simulink library "casper_library_accumulators"  (Simulink 7.0)
values from neighbouring files (symbols this model uses):
  blockCountBits = ceil(log2(numBlocks))    [readback_address_dram_vacc_mask.m]
  blockRowBits = 0    [readback_address_dram_vacc_mask.m]
libraries: xbsIndex_r4 x622, xbsReplacements_r4 x61, casper_library_misc x17, xps_library x9
(part 2 of 5)

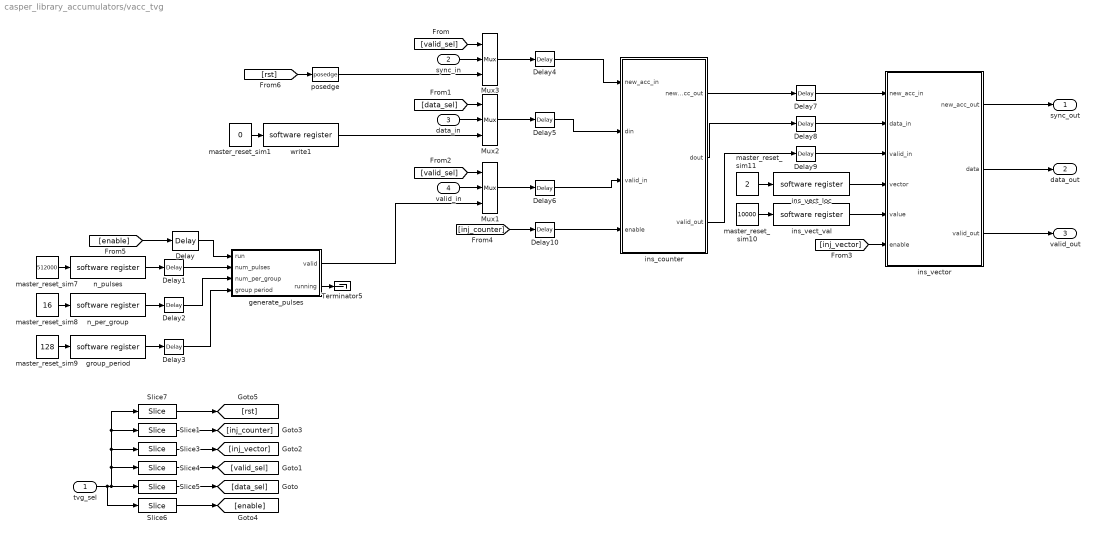
== system casper_library_accumulators/vacc_tvg ==
  tvg_sel : Inport  OutDataType=sfix(16)  OutScaling=2^0
  sync_in : Inport  Port=2  OutDataType=sfix(16)  OutScaling=2^0
  data_in : Inport  Port=3  OutDataType=sfix(16)  OutScaling=2^0
  valid_in : Inport  Port=4  OutDataType=sfix(16)  OutScaling=2^0
  Delay : xbsIndex_r4/Delay  en=off  latency=1  dbl_ovrd=off  reg_retiming=on  block_type=delay
      settings: xl_area=[0, 0, 0, 0, 0, 0, 0]
  Delay{1..10} (10 alike) : xbsIndex_r4/Delay  en=off  latency=2  dbl_ovrd=off  reg_retiming=on  block_type=delay
  Mux1 : xbsIndex_r4/Mux  inputs=2  en=off  latency=0  precision=Full  arith_type="Signed  (2's comp)"  n_bits=8  bin_pt=2  quantization=Truncate  overflow=Wrap  dbl_ovrd=off  block_type=mux
      settings: xl_area=[0, 0, 0, 0, 0, 0, 0]
  Mux2 : xbsIndex_r4/Mux  inputs=2  en=off  latency=0  precision=Full  arith_type="Signed  (2's comp)"  n_bits=8  bin_pt=2  quantization=Truncate  overflow=Wrap  dbl_ovrd=off  block_type=mux
      settings: xl_area=[0, 0, 0, 0, 0, 0, 0]
  Mux3 : xbsIndex_r4/Mux  inputs=2  en=off  latency=0  precision=Full  arith_type="Signed  (2's comp)"  n_bits=8  bin_pt=2  quantization=Truncate  overflow=Wrap  dbl_ovrd=off  block_type=mux
      settings: xl_area=[0, 0, 0, 0, 0, 0, 0]
  Slice1 : xbsIndex_r4/Slice  nbits=1  boolean_output=on  mode=Lower Bit Location + Width  bit1=0  base1=MSB of Input  bit0=4  base0=LSB of Input  dbl_ovrd=off  block_type=slice
      settings: infoedit="Extracts a given range of bits from each input sample and presents it at the output.  The output type is ordinarily unsigned with binary point at zero, but can be Boolean when the slice is one bit wide.<P><P>Hardware notes: In hardware this block costs nothing."  block_version=10.1.3
  Slice3 : xbsIndex_r4/Slice  nbits=1  boolean_output=on  mode=Lower Bit Location + Width  bit1=0  base1=MSB of Input  bit0=3  base0=LSB of Input  dbl_ovrd=off  block_type=slice
      settings: infoedit="Extracts a given range of bits from each input sample and presents it at the output.  The output type is ordinarily unsigned with binary point at zero, but can be Boolean when the slice is one bit wide.<P><P>Hardware notes: In hardware this block costs nothing."  block_version=10.1.3
  Slice4 : xbsIndex_r4/Slice  nbits=1  boolean_output=on  mode=Lower Bit Location + Width  bit1=0  base1=MSB of Input  bit0=2  base0=LSB of Input  dbl_ovrd=off  block_type=slice
      settings: infoedit="Extracts a given range of bits from each input sample and presents it at the output.  The output type is ordinarily unsigned with binary point at zero, but can be Boolean when the slice is one bit wide.<P><P>Hardware notes: In hardware this block costs nothing."  block_version=10.1.3
  Slice5 : xbsIndex_r4/Slice  nbits=1  boolean_output=on  mode=Lower Bit Location + Width  bit1=0  base1=MSB of Input  bit0=1  base0=LSB of Input  dbl_ovrd=off  block_type=slice
      settings: infoedit="Extracts a given range of bits from each input sample and presents it at the output.  The output type is ordinarily unsigned with binary point at zero, but can be Boolean when the slice is one bit wide.<P><P>Hardware notes: In hardware this block costs nothing."  block_version=10.1.3
  Slice6 : xbsIndex_r4/Slice  nbits=1  boolean_output=on  mode=Lower Bit Location + Width  bit1=0  base1=MSB of Input  bit0=0  base0=LSB of Input  dbl_ovrd=off  block_type=slice
      settings: infoedit="Extracts a given range of bits from each input sample and presents it at the output.  The output type is ordinarily unsigned with binary point at zero, but can be Boolean when the slice is one bit wide.<P><P>Hardware notes: In hardware this block costs nothing."  block_version=10.1.3
  Slice7 : xbsIndex_r4/Slice  nbits=1  boolean_output=on  mode=Lower Bit Location + Width  bit1=0  base1=MSB of Input  bit0=5  base0=LSB of Input  dbl_ovrd=off  block_type=slice
      settings: infoedit="Extracts a given range of bits from each input sample and presents it at the output.  The output type is ordinarily unsigned with binary point at zero, but can be Boolean when the slice is one bit wide.<P><P>Hardware notes: In hardware this block costs nothing."  block_version=10.1.3
  Terminator5 : Terminator
  generate_pulses : Subsystem
  group_period : xps_library/software register  Tag=xps:sw_reg  SystemSampleTime=-1  io_dir=From Processor  arith_type=Unsigned  bitwidth=32  bin_pt=0  sample_period=1  gw_name=r_4f_2x_16a_r322m_vacc_tvg0_group_period_user_data_out
      link override qdr_vacc_dram_tvg1_group_period_user_data_out: arith_type=Unsigned  n_bits=32  bin_pt=0  period=1
      link override qdr_vacc_qdr_tvg_group_period_user_data_out: arith_type=Unsigned  n_bits=32  bin_pt=0  period=1
      link override r_4f_2x_16a_r322m_vacc_tvg0_group_period_user_data_out: arith_type=Unsigned  n_bits=32  bin_pt=0  period=1
      link override test_d_v_p_10_1_new_packet_format_qdr_tvg_group_period_user_data_out: arith_type=Unsigned  n_bits=32  bin_pt=0  period=1
      link override test_qdr_vacc2_vacc_tvg_group_period_user_data_out: arith_type=Unsigned  n_bits=32  bin_pt=0  period=1
      link override test_qdr_vacc3_vacc_tvg_group_period_user_data_out: arith_type=Unsigned  n_bits=32  bin_pt=0  period=1
      link override test_qdr_vacc_qdr_tvg_group_period_user_data_out: arith_type=Unsigned  n_bits=32  bin_pt=0  period=1
      link override test_qdr_vacc_vacc_tvg_group_period_user_data_out: arith_type=Unsigned  n_bits=32  bin_pt=0  period=1
      link override test_vacc_10_1_new_pkt_form_qdr_tvg_group_period_user_data_out: arith_type=Unsigned  n_bits=32  bin_pt=0  period=1
      link override test_vacc_pkt_10_1_vacc_tvg0_group_period_user_data_out: arith_type=Unsigned  n_bits=32  bin_pt=0  period=1
      link override test_vacc_pkt_10_1_vacc_tvg_group_period_user_data_out: arith_type=Unsigned  n_bits=32  bin_pt=0  period=1
      link override xflow_sim_8a_vacc_tvg0_group_period_user_data_out: arith_type=Unsigned  n_bits=32  bin_pt=0  period=1
      link override xflow_sim_vacc_tvg0_group_period_user_data_out: arith_type=Unsigned  n_bits=32  bin_pt=0  period=1
  ins_counter : Subsystem  mask{vec_len=len}
      mask prompts: vec_len "Vector Length?"
      mask init:
      | fmtstr = sprintf('Vector Length: %d', vec_len);
      | set_param(gcb, 'AttributesFormatString', fmtstr);
      settings: AttributesFormatString=Vector Length: 139264
  ins_vect_loc : xps_library/software register  Tag=xps:sw_reg  SystemSampleTime=-1  io_dir=From Processor  arith_type=Unsigned  bitwidth=32  bin_pt=0  sample_period=1  gw_name=r_4f_2x_16a_r322m_vacc_tvg0_ins_vect_loc_user_data_out
      link override qdr_vacc_dram_tvg1_inject_vector_location_user_data_out: arith_type=Unsigned  n_bits=32  bin_pt=0  period=1
      link override qdr_vacc_qdr_tvg_inject_vector_location_user_data_out: arith_type=Unsigned  n_bits=32  bin_pt=0  period=1
      link override r_4f_2x_16a_r322m_vacc_tvg0_ins_vect_loc_user_data_out: arith_type=Unsigned  n_bits=32  bin_pt=0  period=1
      link override test_d_v_p_10_1_new_packet_format_qdr_tvg_inject_vector_location_user_data_out: arith_type=Unsigned  n_bits=32  bin_pt=0  period=1
      link override test_qdr_vacc2_vacc_tvg_ins_vect_loc_user_data_out: arith_type=Unsigned  n_bits=32  bin_pt=0  period=1
      link override test_qdr_vacc3_vacc_tvg_ins_vect_loc_user_data_out: arith_type=Unsigned  n_bits=32  bin_pt=0  period=1
      link override test_qdr_vacc_qdr_tvg_inject_vector_location_user_data_out: arith_type=Unsigned  n_bits=32  bin_pt=0  period=1
      link override test_qdr_vacc_vacc_tvg_ins_vect_loc_user_data_out: arith_type=Unsigned  n_bits=32  bin_pt=0  period=1
      link override test_vacc_10_1_new_pkt_form_qdr_tvg_inject_vector_location_user_data_out: arith_type=Unsigned  n_bits=32  bin_pt=0  period=1
      link override test_vacc_pkt_10_1_vacc_tvg0_ins_vect_loc_user_data_out: arith_type=Unsigned  n_bits=32  bin_pt=0  period=1
      link override test_vacc_pkt_10_1_vacc_tvg_inject_vector_location_user_data_out: arith_type=Unsigned  n_bits=32  bin_pt=0  period=1
      link override test_vacc_pkt_10_1_vacc_tvg_ins_vect_loc_user_data_out: arith_type=Unsigned  n_bits=32  bin_pt=0  period=1
      link override xflow_sim_8a_vacc_tvg0_ins_vect_loc_user_data_out: arith_type=Unsigned  n_bits=32  bin_pt=0  period=1
      link override xflow_sim_vacc_tvg0_ins_vect_loc_user_data_out: arith_type=Unsigned  n_bits=32  bin_pt=0  period=1
  ins_vect_val : xps_library/software register  Tag=xps:sw_reg  SystemSampleTime=-1  io_dir=From Processor  arith_type=Unsigned  bitwidth=32  bin_pt=0  sample_period=1  gw_name=r_4f_2x_16a_r322m_vacc_tvg0_ins_vect_val_user_data_out
      link override qdr_vacc_dram_tvg1_inject_vector_value_user_data_out: arith_type=Unsigned  n_bits=32  bin_pt=0  period=1
      link override qdr_vacc_qdr_tvg_inject_vector_value_user_data_out: arith_type=Unsigned  n_bits=32  bin_pt=0  period=1
      link override r_4f_2x_16a_r322m_vacc_tvg0_ins_vect_val_user_data_out: arith_type=Unsigned  n_bits=32  bin_pt=0  period=1
      link override test_d_v_p_10_1_new_packet_format_qdr_tvg_inject_vector_value_user_data_out: arith_type="Signed  (2's comp)"  n_bits=32  bin_pt=0  period=1
      link override test_qdr_vacc2_vacc_tvg_ins_vect_val_user_data_out: arith_type=Unsigned  n_bits=32  bin_pt=0  period=1
      link override test_qdr_vacc3_vacc_tvg_ins_vect_val_user_data_out: arith_type=Unsigned  n_bits=32  bin_pt=0  period=1
      link override test_qdr_vacc_qdr_tvg_inject_vector_value_user_data_out: arith_type="Signed  (2's comp)"  n_bits=32  bin_pt=0  period=1
      link override test_qdr_vacc_vacc_tvg_ins_vect_val_user_data_out: arith_type=Unsigned  n_bits=32  bin_pt=0  period=1
      link override test_vacc_10_1_new_pkt_form_qdr_tvg_inject_vector_value_user_data_out: arith_type="Signed  (2's comp)"  n_bits=32  bin_pt=0  period=1
      link override test_vacc_pkt_10_1_vacc_tvg0_ins_vect_val_user_data_out: arith_type=Unsigned  n_bits=32  bin_pt=0  period=1
      link override test_vacc_pkt_10_1_vacc_tvg_inject_vector_value_user_data_out: arith_type="Signed  (2's comp)"  n_bits=32  bin_pt=0  period=1
      link override test_vacc_pkt_10_1_vacc_tvg_ins_vect_val_user_data_out: arith_type="Signed  (2's comp)"  n_bits=32  bin_pt=0  period=1
      link override xflow_sim_8a_vacc_tvg0_ins_vect_val_user_data_out: arith_type=Unsigned  n_bits=32  bin_pt=0  period=1
      link override xflow_sim_vacc_tvg0_ins_vect_val_user_data_out: arith_type=Unsigned  n_bits=32  bin_pt=0  period=1
  ins_vector : Subsystem  mask{num_vectors=len}
      mask prompts: num_vectors "number of vectors"
      mask init:
      | fmtstr = sprintf('Vector Length: %d', num_vectors);
      | set_param(gcb, 'AttributesFormatString', fmtstr);
      settings: AttributesFormatString=Vector Length: 139264
  master_reset_sim1 : Constant  Value=0  OutDataType=sfix(16)  OutScaling=2^0
  master_reset_sim10 : Constant  Value=10000  OutDataType=sfix(16)  OutScaling=2^0
  master_reset_sim11 : Constant  Value=2  OutDataType=sfix(16)  OutScaling=2^0
  master_reset_sim7 : Constant  Value=512000  OutDataType=sfix(16)  OutScaling=2^0
  master_reset_sim8 : Constant  Value=16  OutDataType=sfix(16)  OutScaling=2^0
  master_reset_sim9 : Constant  Value=128  OutDataType=sfix(16)  OutScaling=2^0
  n_per_group : xps_library/software register  Tag=xps:sw_reg  SystemSampleTime=-1  io_dir=From Processor  arith_type=Unsigned  bitwidth=32  bin_pt=0  sample_period=1  gw_name=r_4f_2x_16a_r322m_vacc_tvg0_n_per_group_user_data_out
      link override qdr_vacc_dram_tvg1_num_per_group_user_data_out: arith_type=Unsigned  n_bits=32  bin_pt=0  period=1
      link override qdr_vacc_qdr_tvg_num_per_group_user_data_out: arith_type=Unsigned  n_bits=32  bin_pt=0  period=1
      link override r_4f_2x_16a_r322m_vacc_tvg0_n_per_group_user_data_out: arith_type=Unsigned  n_bits=32  bin_pt=0  period=1
      link override test_d_v_p_10_1_new_packet_format_qdr_tvg_num_per_group_user_data_out: arith_type=Unsigned  n_bits=32  bin_pt=0  period=1
      link override test_qdr_vacc2_vacc_tvg_n_per_group_user_data_out: arith_type=Unsigned  n_bits=32  bin_pt=0  period=1
      link override test_qdr_vacc3_vacc_tvg_n_per_group_user_data_out: arith_type=Unsigned  n_bits=32  bin_pt=0  period=1
      link override test_qdr_vacc_qdr_tvg_num_per_group_user_data_out: arith_type=Unsigned  n_bits=32  bin_pt=0  period=1
      link override test_qdr_vacc_vacc_tvg_n_per_group_user_data_out: arith_type=Unsigned  n_bits=32  bin_pt=0  period=1
      link override test_vacc_10_1_new_pkt_form_qdr_tvg_num_per_group_user_data_out: arith_type=Unsigned  n_bits=32  bin_pt=0  period=1
      link override test_vacc_pkt_10_1_vacc_tvg0_num_per_group_user_data_out: arith_type=Unsigned  n_bits=32  bin_pt=0  period=1
      link override test_vacc_pkt_10_1_vacc_tvg_num_per_group_user_data_out: arith_type=Unsigned  n_bits=32  bin_pt=0  period=1
      link override xflow_sim_8a_vacc_tvg0_num_per_group_user_data_out: arith_type=Unsigned  n_bits=32  bin_pt=0  period=1
      link override xflow_sim_vacc_tvg0_num_per_group_user_data_out: arith_type=Unsigned  n_bits=32  bin_pt=0  period=1
  n_pulses : xps_library/software register  Tag=xps:sw_reg  SystemSampleTime=-1  io_dir=From Processor  arith_type=Unsigned  bitwidth=32  bin_pt=0  sample_period=1  gw_name=r_4f_2x_16a_r322m_vacc_tvg0_n_pulses_user_data_out
      link override qdr_vacc_dram_tvg1_num_pulses_user_data_out: arith_type=Unsigned  n_bits=32  bin_pt=0  period=1
      link override qdr_vacc_qdr_tvg_num_pulses_user_data_out: arith_type=Unsigned  n_bits=32  bin_pt=0  period=1
      link override r_4f_2x_16a_r322m_vacc_tvg0_n_pulses_user_data_out: arith_type=Unsigned  n_bits=32  bin_pt=0  period=1
      link override test_d_v_p_10_1_new_packet_format_qdr_tvg_num_pulses_user_data_out: arith_type=Unsigned  n_bits=32  bin_pt=0  period=1
      link override test_qdr_vacc2_vacc_tvg_n_pulses_user_data_out: arith_type=Unsigned  n_bits=32  bin_pt=0  period=1
      link override test_qdr_vacc3_vacc_tvg_n_pulses_user_data_out: arith_type=Unsigned  n_bits=32  bin_pt=0  period=1
      link override test_qdr_vacc_qdr_tvg_num_pulses_user_data_out: arith_type=Unsigned  n_bits=32  bin_pt=0  period=1
      link override test_qdr_vacc_vacc_tvg_n_pulses_user_data_out: arith_type=Unsigned  n_bits=32  bin_pt=0  period=1
      link override test_vacc_10_1_new_pkt_form_qdr_tvg_num_pulses_user_data_out: arith_type=Unsigned  n_bits=32  bin_pt=0  period=1
      link override test_vacc_pkt_10_1_vacc_tvg0_num_pulses_user_data_out: arith_type=Unsigned  n_bits=32  bin_pt=0  period=1
      link override test_vacc_pkt_10_1_vacc_tvg_num_pulses_user_data_out: arith_type=Unsigned  n_bits=32  bin_pt=0  period=1
      link override xflow_sim_8a_vacc_tvg0_num_pulses_user_data_out: arith_type=Unsigned  n_bits=32  bin_pt=0  period=1
      link override xflow_sim_vacc_tvg0_num_pulses_user_data_out: arith_type=Unsigned  n_bits=32  bin_pt=0  period=1
  posedge : casper_library_misc/posedge  Tag=Rising Edge Detector  SystemSampleTime=-1
  write1 : xps_library/software register  Tag=xps:sw_reg  SystemSampleTime=-1  io_dir=From Processor  arith_type=Unsigned  bitwidth=32  bin_pt=0  sample_period=1  gw_name=r_4f_2x_16a_r322m_vacc_tvg0_write1_user_data_out
      link override qdr_vacc_dram_tvg1_write1_user_data_out: arith_type=Unsigned  n_bits=32  bin_pt=0  period=1
      link override qdr_vacc_qdr_tvg_write1_user_data_out: arith_type=Unsigned  n_bits=32  bin_pt=0  period=1
      link override r_4f_2x_16a_r322m_vacc_tvg0_write1_user_data_out: arith_type=Unsigned  n_bits=32  bin_pt=0  period=1
      link override test_d_v_p_10_1_new_packet_format_qdr_tvg_write1_user_data_out: arith_type="Signed  (2's comp)"  n_bits=32  bin_pt=0  period=1
      link override test_qdr_vacc2_vacc_tvg_write1_user_data_out: arith_type=Unsigned  n_bits=32  bin_pt=0  period=1
      link override test_qdr_vacc3_vacc_tvg_write1_user_data_out: arith_type=Unsigned  n_bits=32  bin_pt=0  period=1
      link override test_qdr_vacc_qdr_tvg_write1_user_data_out: arith_type="Signed  (2's comp)"  n_bits=32  bin_pt=0  period=1
      link override test_qdr_vacc_vacc_tvg_write1_user_data_out: arith_type=Unsigned  n_bits=32  bin_pt=0  period=1
      link override test_vacc_10_1_new_pkt_form_qdr_tvg_write1_user_data_out: arith_type="Signed  (2's comp)"  n_bits=32  bin_pt=0  period=1
      link override test_vacc_pkt_10_1_vacc_tvg0_write1_user_data_out: arith_type=Unsigned  n_bits=32  bin_pt=0  period=1
      link override test_vacc_pkt_10_1_vacc_tvg_write1_user_data_out: arith_type="Signed  (2's comp)"  n_bits=32  bin_pt=0  period=1
      link override xflow_sim_8a_vacc_tvg0_write1_user_data_out: arith_type=Unsigned  n_bits=32  bin_pt=0  period=1
      link override xflow_sim_vacc_tvg0_write1_user_data_out: arith_type=Unsigned  n_bits=32  bin_pt=0  period=1
  sync_out : Outport  OutDataType=sfix(16)  OutScaling=2^0
  data_out : Outport  Port=2  OutDataType=sfix(16)  OutScaling=2^0
  valid_out : Outport  Port=3  OutDataType=sfix(16)  OutScaling=2^0
  wires:
  Delay10/1 -> ins_counter/4(enable)
  Delay9/1 -> ins_vector/3(valid_in)
  Delay8/1 -> ins_vector/2(data_in)
  Delay7/1 -> ins_vector/1(new_acc_in)
  Delay6/1 -> ins_counter/3(valid_in)
  Delay5/1 -> ins_counter/2(din)
  Delay4/1 -> ins_counter/1(new_acc_in)
  Delay3/1 -> generate_pulses/4(group period)
  Delay2/1 -> generate_pulses/3(num_per_group)
  Delay1/1 -> generate_pulses/2(num_pulses)
  write1/1 -> Mux2/3
  master_reset_sim1/1 -> write1/1
  [rst] -> posedge/1
  n_pulses/1 -> Delay1/1
  master_reset_sim7/1 -> n_pulses/1
  n_per_group/1 -> Delay2/1
  master_reset_sim8/1 -> n_per_group/1
  group_period/1 -> Delay3/1
  master_reset_sim9/1 -> group_period/1
  Mux1/1 -> Delay6/1
  valid_in/1 -> Mux1/2
  ins_vector/1(new_acc_out) -> sync_out/1
  ins_vector/2(data) -> data_out/1
  ins_vector/3(valid_out) -> valid_out/1
  ins_counter/1(new_acc_out) -> Delay7/1
  Mux2/1 -> Delay5/1
  data_in/1 -> Mux2/2
  sync_in/1 -> Mux3/2
  Mux3/1 -> Delay4/1
  Slice5/1 -> [data_sel]
  tvg_sel/1 -> Slice5/1, Slice3/1, Slice1/1, Slice7/1, Slice4/1, Slice6/1
  Slice4/1 -> [valid_sel]
  [valid_sel] -> Mux3/1
  [data_sel] -> Mux2/1
  [valid_sel] -> Mux1/1
  Slice3/1 -> [inj_vector]
  Slice1/1 -> [inj_counter]
  [enable] -> Delay/1
  ins_counter/2(dout) -> Delay8/1
  ins_counter/3(valid_out) -> Delay9/1
  generate_pulses/1(valid) -> Mux1/3
  posedge/1 -> Mux3/3
  [inj_vector] -> ins_vector/6(enable)
  master_reset_sim11/1 -> ins_vect_loc/1
  ins_vect_loc/1 -> ins_vector/4(vector)
  master_reset_sim10/1 -> ins_vect_val/1
  ins_vect_val/1 -> ins_vector/5(value)
  [inj_counter] -> Delay10/1
  Slice6/1 -> [enable]
  Slice7/1 -> [rst]
  Delay/1 -> generate_pulses/1(run)
  generate_pulses/2(running) -> Terminator5/1

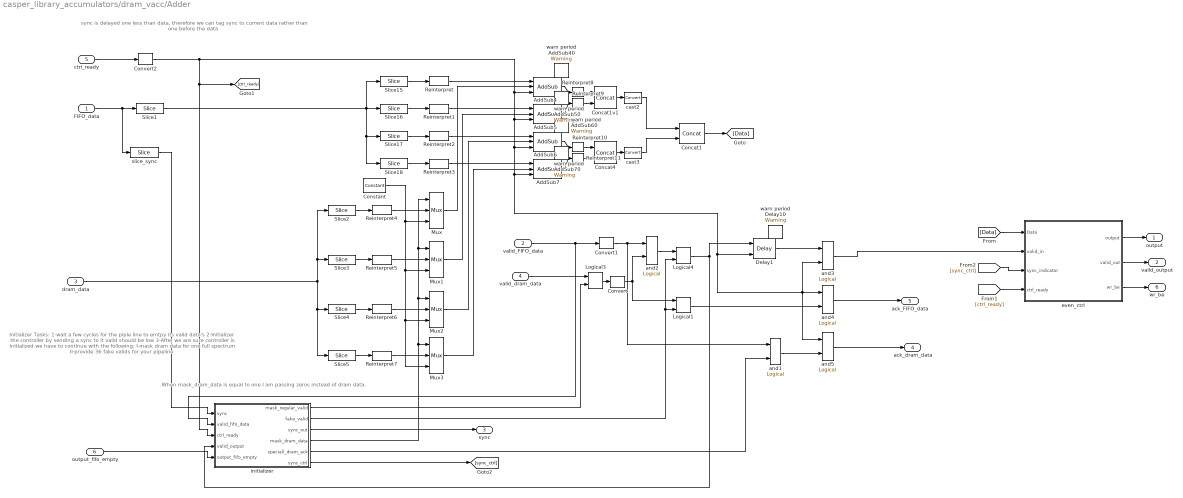
== system casper_library_accumulators/dram_vacc/Adder ==
  note: When mask_dram_data is equal to one
      | I am passing zeros instead of dram data.
  note: Initializer Tasks:
      | 1-wait a few cycles for the piple line to emtpy
      | its valid data's
      | 2-Initializer the controller by sending a sync to it
      | valid should be low
      | 3-After we are sure controller is initialized we have to
      | continue with the following:
      | I-mask dram data for one full spectrum
      | II-provide 36 fake valids for your pipeline
  note: sync is delayed one less than data,
      | therefore we can tag sync to current data rather than
      | one before the data
  FIFO_data : Inport  OutDataType=sfix(16)  OutScaling=2^0
  valid_FIFO_data : Inport  Port=2  OutDataType=sfix(16)  OutScaling=2^0
  dram_data : Inport  Port=3  OutDataType=sfix(16)  OutScaling=2^0
  valid_dram_data : Inport  Port=4  OutDataType=sfix(16)  OutScaling=2^0
  ctrl_ready : Inport  Port=5  OutDataType=sfix(16)  OutScaling=2^0
  output_fifo_empty : Inport  Port=6  OutDataType=sfix(16)  OutScaling=2^0
  AddSub{4..7} (4 alike) : xbsIndex_r4/AddSub  mode=Addition  use_carryin=off  use_carryout=off  en=on  latency=3  precision=User Defined  arith_type="Signed  (2's comp)"  n_bits=32  bin_pt=0  quantization="Round  (unbiased: +/- Inf)"  overflow=Wrap  dbl_ovrd=off  use_behavioral_HDL=on  pipelined=on  use_rpm=on  block_type=addsub
      settings: xl_area=[0, 0, 0, 0, 0, 0, 0]  block_version=9.2.01
  Concat1 : xbsIndex_r4/Concat  num_inputs=2  dbl_ovrd=off  block_type=concat
      settings: block_version=9.2.01
  Concat1v1 : xbsIndex_r4/Concat  num_inputs=2  dbl_ovrd=off  block_type=concat
      settings: block_version=9.2.01
  Concat4 : xbsIndex_r4/Concat  num_inputs=2  dbl_ovrd=off  block_type=concat
      settings: block_version=9.2.01
  Constant : xbsIndex_r4/Constant  arith_type=Signed (2's comp)  const=0  n_bits=32  bin_pt=0  explicit_period=on  period=1  equ=P=C  opselect=C  inp2=PCIN>>17  opr=+  inp1=P  carry=CIN  dbl_ovrd=off  block_type=constant
      settings: block_version=9.2.01
  Convert : xbsIndex_r4/Convert  arith_type=Boolean  n_bits=8  bin_pt=6  quantization=Truncate  overflow=Wrap  latency=0  dbl_ovrd=off  pipeline=off  block_type=convert
      settings: xl_area=[0, 0, 0, 0, 0, 0, 0]  block_version=9.2.01
  Convert1 : xbsIndex_r4/Convert  arith_type=Boolean  n_bits=8  bin_pt=6  quantization=Truncate  overflow=Wrap  latency=0  dbl_ovrd=off  pipeline=off  block_type=convert
      settings: xl_area=[0, 0, 0, 0, 0, 0, 0]  block_version=9.2.01
  Convert2 : xbsIndex_r4/Convert  arith_type=Boolean  n_bits=8  bin_pt=6  quantization=Truncate  overflow=Wrap  latency=0  dbl_ovrd=off  pipeline=off  block_type=convert
      settings: xl_area=[0, 0, 0, 0, 0, 0, 0]  block_version=9.2.01
  Delay1 : xbsIndex_r4/Delay  en=on  latency=3  dbl_ovrd=off  reg_retiming=off  block_type=delay
      settings: xl_area=[0, 0, 0, 0, 0, 0, 0]  block_version=9.2.01
  Logical1 : xbsIndex_r4/Logical  logical_function=OR  inputs=2  en=off  latency=0  precision=Full  arith_type=Unsigned  n_bits=8  bin_pt=2  align_bp=on  dbl_ovrd=off  block_type=logical
      settings: xl_area=[0, 0, 0, 0, 0, 0, 0]  block_version=9.2.01
  Logical3 : xbsIndex_r4/Logical  logical_function=AND  inputs=2  en=off  latency=0  precision=Full  arith_type=Unsigned  n_bits=8  bin_pt=2  align_bp=on  dbl_ovrd=off  block_type=logical
      settings: xl_area=[0, 0, 0, 0, 0, 0, 0]  block_version=9.2.01
  Logical4 : xbsIndex_r4/Logical  logical_function=OR  inputs=2  en=off  latency=0  precision=Full  arith_type=Unsigned  n_bits=8  bin_pt=2  align_bp=on  dbl_ovrd=off  block_type=logical
      settings: xl_area=[0, 0, 0, 0, 0, 0, 0]  block_version=9.2.01
  Mux{,1..3} (4 alike) : xbsIndex_r4/Mux  inputs=2  en=off  latency=0  precision=Full  arith_type="Signed  (2's comp)"  n_bits=8  bin_pt=2  quantization=Truncate  overflow=Wrap  dbl_ovrd=off  block_type=mux
      settings: xl_area=[0, 0, 0, 0, 0, 0, 0]  block_version=9.2.01
  Reinterpret{,1..7} (8 alike) : xbsIndex_r4/Reinterpret  force_arith_type=on  arith_type="Signed  (2's comp)"  force_bin_pt=on  bin_pt=0  block_type=reinterpret
      settings: infoedit="Changes signal type without altering the binary representation.   You can changed the signal between signed and unsigned, and relocate the binary point.<P><P>Hardware notes: In hardware this block costs nothing.<P><P>Example:  Suppose the input is 6 bits wide, signed, with 2 fractional bits, and the output is forced to unsigned with 0 fractional bits.  Then an input of -2.0 (1110.00 in binary 2's complement) becomes an output of 56 (111000 in binary)."  block_version=9.2.01
  Reinterpret{8..11} (4 alike) : xbsIndex_r4/Reinterpret  force_arith_type=on  arith_type=Unsigned  force_bin_pt=on  bin_pt=0  block_type=reinterpret
      settings: infoedit="Changes signal type without altering the binary representation.   You can changed the signal between signed and unsigned, and relocate the binary point.<P><P>Hardware notes: In hardware this block costs nothing.<P><P>Example:  Suppose the input is 6 bits wide, signed, with 2 fractional bits, and the output is forced to unsigned with 0 fractional bits.  Then an input of -2.0 (1110.00 in binary 2's complement) becomes an output of 56 (111000 in binary)."  block_version=9.2.01
  Slice1 : xbsIndex_r4/Slice  nbits=128  boolean_output=off  mode=Lower Bit Location + Width  bit1=0  base1=MSB of Input  bit0=0  base0=LSB of Input  dbl_ovrd=off  block_type=slice
      settings: infoedit="Extracts a given range of bits from each input sample and presents it at the output.  The output type is ordinarily unsigned with binary point at zero, but can be Boolean when the slice is one bit wide.<P><P>Hardware notes: In hardware this block costs nothing."  block_version=9.2.01
  Slice15 : xbsIndex_r4/Slice  nbits=32  boolean_output=off  mode=Lower Bit Location + Width  bit1=96  base1=MSB of Input  bit0=96  base0=LSB of Input  dbl_ovrd=off  block_type=slice
      settings: infoedit="Extracts a given range of bits from each input sample and presents it at the output.  The output type is ordinarily unsigned with binary point at zero, but can be Boolean when the slice is one bit wide.<P><P>Hardware notes: In hardware this block costs nothing."  block_version=9.2.01
  Slice16 : xbsIndex_r4/Slice  nbits=32  boolean_output=off  mode=Lower Bit Location + Width  bit1=-32  base1=MSB of Input  bit0=64  base0=LSB of Input  dbl_ovrd=off  block_type=slice
      settings: infoedit="Extracts a given range of bits from each input sample and presents it at the output.  The output type is ordinarily unsigned with binary point at zero, but can be Boolean when the slice is one bit wide.<P><P>Hardware notes: In hardware this block costs nothing."  block_version=9.2.01
  Slice17 : xbsIndex_r4/Slice  nbits=32  boolean_output=off  mode=Lower Bit Location + Width  bit1=0  base1=MSB of Input  bit0=32  base0=LSB of Input  dbl_ovrd=off  block_type=slice
      settings: infoedit="Extracts a given range of bits from each input sample and presents it at the output.  The output type is ordinarily unsigned with binary point at zero, but can be Boolean when the slice is one bit wide.<P><P>Hardware notes: In hardware this block costs nothing."  block_version=9.2.01
  Slice18 : xbsIndex_r4/Slice  nbits=32  boolean_output=off  mode=Lower Bit Location + Width  bit1=0  base1=MSB of Input  bit0=0  base0=LSB of Input  dbl_ovrd=off  block_type=slice
      settings: infoedit="Extracts a given range of bits from each input sample and presents it at the output.  The output type is ordinarily unsigned with binary point at zero, but can be Boolean when the slice is one bit wide.<P><P>Hardware notes: In hardware this block costs nothing."  block_version=9.2.01
  Slice2 : xbsIndex_r4/Slice  nbits=32  boolean_output=off  mode=Lower Bit Location + Width  bit1=0  base1=MSB of Input  bit0=104  base0=LSB of Input  dbl_ovrd=off  block_type=slice
      settings: infoedit="Extracts a given range of bits from each input sample and presents it at the output.  The output type is ordinarily unsigned with binary point at zero, but can be Boolean when the slice is one bit wide.<P><P>Hardware notes: In hardware this block costs nothing."  block_version=9.2.01
  Slice3 : xbsIndex_r4/Slice  nbits=32  boolean_output=off  mode=Lower Bit Location + Width  bit1=72  base1=MSB of Input  bit0=72  base0=LSB of Input  dbl_ovrd=off  block_type=slice
      settings: infoedit="Extracts a given range of bits from each input sample and presents it at the output.  The output type is ordinarily unsigned with binary point at zero, but can be Boolean when the slice is one bit wide.<P><P>Hardware notes: In hardware this block costs nothing."  block_version=9.2.01
  Slice4 : xbsIndex_r4/Slice  nbits=32  boolean_output=off  mode=Lower Bit Location + Width  bit1=0  base1=MSB of Input  bit0=32  base0=LSB of Input  dbl_ovrd=off  block_type=slice
      settings: infoedit="Extracts a given range of bits from each input sample and presents it at the output.  The output type is ordinarily unsigned with binary point at zero, but can be Boolean when the slice is one bit wide.<P><P>Hardware notes: In hardware this block costs nothing."  block_version=9.2.01
  Slice5 : xbsIndex_r4/Slice  nbits=32  boolean_output=off  mode=Lower Bit Location + Width  bit1=0  base1=MSB of Input  bit0=0  base0=LSB of Input  dbl_ovrd=off  block_type=slice
      settings: infoedit="Extracts a given range of bits from each input sample and presents it at the output.  The output type is ordinarily unsigned with binary point at zero, but can be Boolean when the slice is one bit wide.<P><P>Hardware notes: In hardware this block costs nothing."  block_version=9.2.01
  and1 : xbsIndex_r4/Logical  logical_function=OR  inputs=2  en=off  latency=0  precision=Full  arith_type=Unsigned  n_bits=8  bin_pt=2  align_bp=on  dbl_ovrd=off  block_type=logical
      settings: xl_area=[0, 0, 0, 0, 0, 0, 0]  block_version=9.2.01
  and{2..5} (4 alike) : xbsIndex_r4/Logical  logical_function=AND  inputs=2  en=off  latency=0  precision=Full  arith_type=Unsigned  n_bits=8  bin_pt=2  align_bp=on  dbl_ovrd=off  block_type=logical
      settings: xl_area=[0, 0, 0, 0, 0, 0, 0]  block_version=9.2.01
  cast2 : xbsIndex_r4/Convert  arith_type=Unsigned  n_bits=72  bin_pt=0  quantization=Truncate  overflow=Wrap  latency=0  dbl_ovrd=off  pipeline=off  block_type=convert
      settings: xl_area=[0, 0, 0, 0, 0, 0, 0]  block_version=9.2.01
  cast3 : xbsIndex_r4/Convert  arith_type=Unsigned  n_bits=72  bin_pt=0  quantization=Truncate  overflow=Wrap  latency=0  dbl_ovrd=off  pipeline=off  block_type=convert
      settings: xl_area=[0, 0, 0, 0, 0, 0, 0]  block_version=9.2.01
  even_ctrl : Subsystem
  initializer : Subsystem
  slice_sync : xbsIndex_r4/Slice  nbits=1  boolean_output=on  mode=Upper Bit Location + Width  bit1=0  base1=MSB of Input  bit0=0  base0=LSB of Input  dbl_ovrd=off  block_type=slice
      settings: infoedit="Extracts a given range of bits from each input sample and presents it at the output.  The output type is ordinarily unsigned with binary point at zero, but can be Boolean when the slice is one bit wide.<P><P>Hardware notes: In hardware this block costs nothing."  block_version=9.2.01
  warn period AddSub{40,50,60,70} (4 alike) : xbsReplacements_r4/Warning  SystemSampleTime=-1  period=1
  warn period Delay10 : xbsReplacements_r4/Warning  SystemSampleTime=-1  period=1
  output : Outport  OutDataType=sfix(16)  OutScaling=2^0
  valid_output : Outport  Port=2  OutDataType=sfix(16)  OutScaling=2^0
  sync : Outport  Port=3  OutDataType=sfix(16)  OutScaling=2^0
  ack_dram_data : Outport  Port=4  OutDataType=sfix(16)  OutScaling=2^0
  ack_FIFO_data : Outport  Port=5  OutDataType=sfix(16)  OutScaling=2^0
  wr_be : Outport  Port=6  OutDataType=sfix(16)  OutScaling=2^0
  wires:
  Reinterpret11/1 -> Concat4/2
  Reinterpret10/1 -> Concat4/1
  Reinterpret9/1 -> Concat1v1/2
  Reinterpret8/1 -> Concat1v1/1
  Reinterpret7/1 -> Mux3/2
  Reinterpret6/1 -> Mux2/2
  Reinterpret5/1 -> Mux1/2
  Reinterpret4/1 -> Mux/2
  Reinterpret3/1 -> AddSub7/1
  Reinterpret2/1 -> AddSub6/1
  Reinterpret1/1 -> AddSub5/1
  Reinterpret/1 -> AddSub4/1
  Logical1/1 -> and4/2
  and1/1 -> and5/2
  and5/1 -> ack_dram_data/1
  Logical4/1 -> initializer/4(valid_output), Delay1/1
  initializer/5(speciall_dram_ack) -> and1/2
  output_fifo_empty/1 -> initializer/5(output_fifo_empty)
  Constant/1 -> Mux2/3, Mux3/3, Mux1/3, Mux/3
  initializer/4(mask_dram_data) -> Mux3/1, Mux2/1, Mux1/1, Mux/1
  Slice2/1 -> Reinterpret4/1
  Slice3/1 -> Reinterpret5/1
  Slice4/1 -> Reinterpret6/1
  Slice5/1 -> Reinterpret7/1
  initializer/3(sync_out) -> sync/1
  and2/1 -> Logical4/1
  and4/1 -> ack_FIFO_data/1
  Delay1/1 -> and3/1
  initializer/2(fake_valid) -> Logical1/2, Logical4/2
  Logical3/1 -> Convert/1
  initializer/1(mask_regular_valid) -> Logical3/2
  valid_dram_data/1 -> Logical3/1
  and3/1 -> even_ctrl/2(valid_in)
  Convert2/1 -> [ctrl_ready], initializer/3(ctrl_ready), AddSub4/3, AddSub5/3, Delay1/2, and5/1, and4/1, and3/2, AddSub7/3, AddSub6/3
  Convert1/1 -> and1/1, and2/1
  Convert/1 -> Logical1/1, and2/2
  slice_sync/1 -> initializer/1(sync)
  Slice1/1 -> Slice18/1, Slice17/1, Slice16/1, Slice15/1
  dram_data/1 -> Slice4/1, Slice5/1, Slice3/1, Slice2/1
  valid_FIFO_data/1 -> Convert1/1, initializer/2(valid_fifo_data)
  ctrl_ready/1 -> Convert2/1
  FIFO_data/1 -> slice_sync/1, Slice1/1
  cast3/1 -> Concat1/2
  Concat4/1 -> cast3/1
  cast2/1 -> Concat1/1
  Concat1v1/1 -> cast2/1
  AddSub7/1 -> Reinterpret11/1
  AddSub6/1 -> Reinterpret10/1
  AddSub5/1 -> Reinterpret9/1
  AddSub4/1 -> Reinterpret8/1
  Mux3/1 -> AddSub7/2
  Mux2/1 -> AddSub6/2
  Mux1/1 -> AddSub5/2
  Mux/1 -> AddSub4/2
  Slice18/1 -> Reinterpret3/1
  Slice17/1 -> Reinterpret2/1
  Slice16/1 -> Reinterpret1/1
  Slice15/1 -> Reinterpret/1
  even_ctrl/1(output) -> output/1
  even_ctrl/2(valid_out) -> valid_output/1
  Concat1/1 -> [Data]
  [Data] -> even_ctrl/1(Data)
  [ctrl_ready] -> even_ctrl/4(ctrl_ready)
  even_ctrl/3(wr_be) -> wr_be/1
  initializer/6(sync_ctrl) -> [sync_ctrl]
  [sync_ctrl] -> even_ctrl/3(sync_indicator)

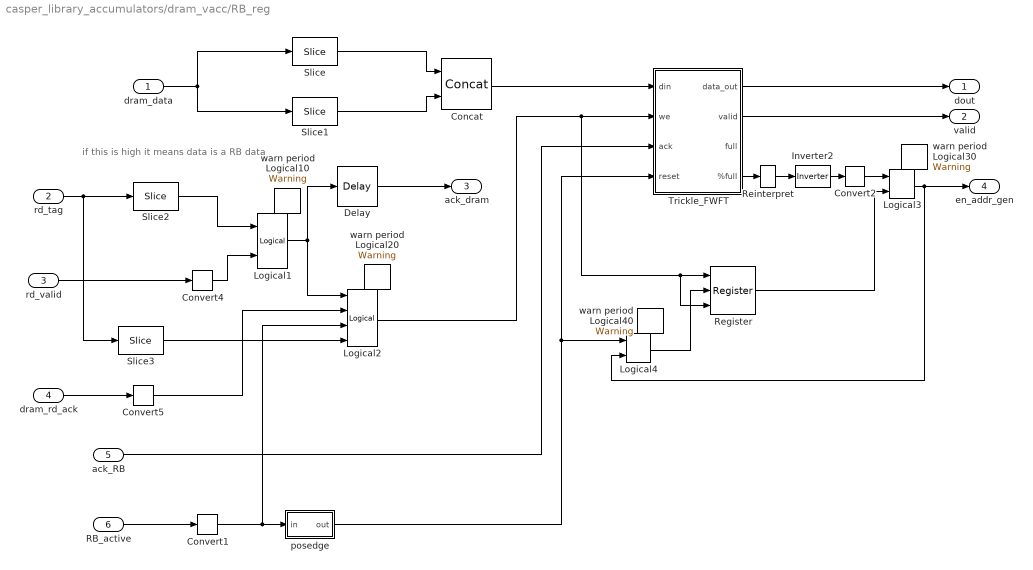
== system casper_library_accumulators/dram_vacc/RB_reg ==
  note: if this is high it means data is a RB data
  dram_data : Inport  OutDataType=sfix(16)  OutScaling=2^0
  rd_tag : Inport  Port=2  OutDataType=sfix(16)  OutScaling=2^0
  rd_valid : Inport  Port=3  OutDataType=sfix(16)  OutScaling=2^0
  dram_rd_ack : Inport  Port=4  OutDataType=sfix(16)  OutScaling=2^0
  ack_RB : Inport  Port=5  OutDataType=sfix(16)  OutScaling=2^0
  RB_active : Inport  Port=6  OutDataType=sfix(16)  OutScaling=2^0
  Concat : xbsIndex_r4/Concat  num_inputs=2  dbl_ovrd=off  block_type=concat
      settings: block_version=9.2.01
  Convert{1..2,4..5} (4 alike) : xbsIndex_r4/Convert  arith_type=Boolean  n_bits=31  bin_pt=0  quantization=Truncate  overflow=Wrap  latency=0  dbl_ovrd=off  pipeline=off  block_type=convert
      settings: xl_area=[0, 0, 0, 0, 0, 0, 0]  block_version=9.2.01
  Delay : xbsIndex_r4/Delay  en=off  latency=1  dbl_ovrd=off  reg_retiming=on  block_type=delay
      settings: xl_area=[0, 0, 0, 0, 0, 0, 0]  block_version=9.2.01
  Inverter2 : xbsIndex_r4/Inverter  en=off  latency=0  dbl_ovrd=off  block_type=inv
      settings: xl_area=[0, 0, 0, 0, 0, 0, 0]  block_version=9.2.01
  Logical1 : xbsIndex_r4/Logical  logical_function=AND  inputs=2  en=off  latency=0  precision=Full  arith_type=Unsigned  n_bits=8  bin_pt=2  align_bp=on  dbl_ovrd=off  block_type=logical
      settings: xl_area=[0, 0, 0, 0, 0, 0, 0]  block_version=9.2.01
  Logical2 : xbsIndex_r4/Logical  logical_function=AND  inputs=4  en=off  latency=0  precision=Full  arith_type=Unsigned  n_bits=8  bin_pt=2  align_bp=on  dbl_ovrd=off  block_type=logical
      settings: xl_area=[0, 0, 0, 0, 0, 0, 0]  block_version=9.2.01
  Logical3 : xbsIndex_r4/Logical  logical_function=AND  inputs=2  en=off  latency=0  precision=Full  arith_type=Unsigned  n_bits=8  bin_pt=2  align_bp=on  dbl_ovrd=off  block_type=logical
      settings: xl_area=[0, 0, 0, 0, 0, 0, 0]  block_version=9.2.01
  Logical4 : xbsIndex_r4/Logical  logical_function=OR  inputs=2  en=off  latency=0  precision=Full  arith_type=Unsigned  n_bits=8  bin_pt=2  align_bp=on  dbl_ovrd=off  block_type=logical
      settings: xl_area=[0, 0, 0, 0, 0, 0, 0]  block_version=9.2.01
  Register : xbsIndex_r4/Register  init=0  rst=on  en=on  dbl_ovrd=off  block_type=register
      settings: xl_area=[0, 0, 0, 0, 0, 0, 0]  block_version=9.2.01
  Reinterpret : xbsIndex_r4/Reinterpret  force_arith_type=on  arith_type=Unsigned  force_bin_pt=on  bin_pt=0  block_type=reinterpret
      settings: infoedit="Changes signal type without altering the binary representation.   You can changed the signal between signed and unsigned, and relocate the binary point.<P><P>Hardware notes: In hardware this block costs nothing.<P><P>Example:  Suppose the input is 6 bits wide, signed, with 2 fractional bits, and the output is forced to unsigned with 0 fractional bits.  Then an input of -2.0 (1110.00 in binary 2's complement) becomes an output of 56 (111000 in binary)."  block_version=9.2.01
  Slice : xbsIndex_r4/Slice  nbits=64  boolean_output=off  mode=Lower Bit Location + Width  bit1=0  base1=MSB of Input  bit0=72  base0=LSB of Input  dbl_ovrd=off  block_type=slice
      settings: infoedit="Extracts a given range of bits from each input sample and presents it at the output.  The output type is ordinarily unsigned with binary point at zero, but can be Boolean when the slice is one bit wide.<P><P>Hardware notes: In hardware this block costs nothing."  block_version=9.2.01
  Slice1 : xbsIndex_r4/Slice  nbits=64  boolean_output=off  mode=Lower Bit Location + Width  bit1=0  base1=MSB of Input  bit0=0  base0=LSB of Input  dbl_ovrd=off  block_type=slice
      settings: infoedit="Extracts a given range of bits from each input sample and presents it at the output.  The output type is ordinarily unsigned with binary point at zero, but can be Boolean when the slice is one bit wide.<P><P>Hardware notes: In hardware this block costs nothing."  block_version=9.2.01
  Slice2 : xbsIndex_r4/Slice  nbits=1  boolean_output=on  mode=Upper Bit Location + Width  bit1=0  base1=MSB of Input  bit0=74  base0=LSB of Input  dbl_ovrd=off  block_type=slice
      settings: infoedit="Extracts a given range of bits from each input sample and presents it at the output.  The output type is ordinarily unsigned with binary point at zero, but can be Boolean when the slice is one bit wide.<P><P>Hardware notes: In hardware this block costs nothing."  block_version=9.2.01
  Slice3 : xbsIndex_r4/Slice  nbits=1  boolean_output=on  mode=Lower Bit Location + Width  bit1=0  base1=MSB of Input  bit0=0  base0=LSB of Input  dbl_ovrd=off  block_type=slice
      settings: infoedit="Extracts a given range of bits from each input sample and presents it at the output.  The output type is ordinarily unsigned with binary point at zero, but can be Boolean when the slice is one bit wide.<P><P>Hardware notes: In hardware this block costs nothing."  block_version=9.2.01
  Trickle_FWFT : Subsystem  mask{depth=16}
      mask init:
      | cursys = gcb ; 
      | set_param([cursys, '/FIFO'], 'depth', depth);
      mask StyleString: popup(16|32|64|128|256|512|1K|2K|4K|8K|16K|32K|64K)
  posedge : Subsystem
  warn period Logical{10,20,30,40} (4 alike) : xbsReplacements_r4/Warning  SystemSampleTime=-1  period=1
  dout : Outport  OutDataType=sfix(16)  OutScaling=2^0
  valid : Outport  Port=2  OutDataType=sfix(16)  OutScaling=2^0
  ack_dram : Outport  Port=3  OutDataType=sfix(16)  OutScaling=2^0
  en_addr_gen : Outport  Port=4  OutDataType=sfix(16)  OutScaling=2^0
  wires:
  Reinterpret/1 -> Inverter2/1
  Convert2/1 -> Logical3/1
  Slice3/1 -> Logical2/4
  Slice2/1 -> Logical1/1
  Convert4/1 -> Logical1/2
  Logical4/1 -> Register/2
  Register/1 -> Logical3/2
  Logical3/1 -> Logical4/2, en_addr_gen/1
  Inverter2/1 -> Convert2/1
  Trickle_FWFT/4(%full) -> Reinterpret/1
  Trickle_FWFT/2(valid) -> valid/1
  Trickle_FWFT/1(data_out) -> dout/1
  posedge/1(out) -> Logical4/1, Trickle_FWFT/4(reset)
  Concat/1 -> Trickle_FWFT/1(din)
  ack_RB/1 -> Trickle_FWFT/3(ack)
  Convert1/1 -> Logical2/3, posedge/1(in)
  dram_data/1 -> Slice1/1, Slice/1
  Slice1/1 -> Concat/2
  Slice/1 -> Concat/1
  Convert5/1 -> Logical2/2
  RB_active/1 -> Convert1/1
  Logical2/1 -> Register/3, Register/1, Trickle_FWFT/2(we)
  dram_rd_ack/1 -> Convert5/1
  Logical1/1 -> Logical2/1, Delay/1
  Delay/1 -> ack_dram/1
  rd_valid/1 -> Convert4/1
  rd_tag/1 -> Slice3/1, Slice2/1

== system casper_library_accumulators/dram_vacc/Trickle_FWFT ==
  note: We needed a FIFO which brings the valid data automatically to the output.
      | The regular XILINX Fifos are not FWFT (First Word Fall Through).
      | We tried to make one but it was really hard to make one agreeing with the exact specs.
      | This module which we have named it Trickle_FWFT Fifo works very similiarly with minor
      | differences which servers our purpose here in the DRAM VACC module.
  note: The real depth of this module is depth+1.
      | The valid signal will go high with one cycle delay.
  din : Inport  OutDataType=sfix(16)  OutScaling=2^0
  we : Inport  Port=2  OutDataType=sfix(16)  OutScaling=2^0
  ack : Inport  Port=3  OutDataType=sfix(16)  OutScaling=2^0
  reset : Inport  Port=4  OutDataType=sfix(16)  OutScaling=2^0
  Convert : xbsIndex_r4/Convert  arith_type=Boolean  n_bits=8  bin_pt=6  quantization=Truncate  overflow=Wrap  latency=0  dbl_ovrd=off  pipeline=off  block_type=convert
      settings: xl_area=[0, 0, 0, 0, 0, 0, 0]  block_version=9.2.01
  Convert1 : xbsIndex_r4/Convert  arith_type=Boolean  n_bits=8  bin_pt=6  quantization=Truncate  overflow=Wrap  latency=0  dbl_ovrd=off  pipeline=off  block_type=convert
      settings: xl_area=[0, 0, 0, 0, 0, 0, 0]  block_version=9.2.01
  Convert2 : xbsIndex_r4/Convert  arith_type=Boolean  n_bits=8  bin_pt=6  quantization=Truncate  overflow=Wrap  latency=0  dbl_ovrd=off  pipeline=off  block_type=convert
      settings: xl_area=[0, 0, 0, 0, 0, 0, 0]  block_version=9.2.01
  FIFO : xbsIndex_r4/FIFO  depth=512  percent_nbits=1  rst=on  en=off  use_dcount=off  use_almost_empty=off  almost_empty_thresh=2  use_almost_full=off  almost_full_thresh=14  dbl_ovrd=off  mem_type=Block RAM  explicit_period=on  period=1  block_type=fifo
      settings: xl_area=[0, 0, 0, 0, 0, 0, 0]  block_version=9.2.01
  Inverter3 : xbsIndex_r4/Inverter  en=off  latency=0  dbl_ovrd=off  block_type=inv
      settings: xl_area=[0, 0, 0, 0, 0, 0, 0]  block_version=9.2.01
  Logical2 : xbsIndex_r4/Logical  logical_function=OR  inputs=2  en=off  latency=0  precision=Full  arith_type=Unsigned  n_bits=8  bin_pt=2  align_bp=on  dbl_ovrd=off  block_type=logical
      settings: xl_area=[0, 0, 0, 0, 0, 0, 0]  block_version=9.2.01
  not_valid : xbsIndex_r4/Register  init=1  rst=on  en=on  dbl_ovrd=off  block_type=register
      settings: xl_area=[0, 0, 0, 0, 0, 0, 0]  block_version=9.2.01
  warn period Convert0 : xbsReplacements_r4/Warning  SystemSampleTime=-1  period=1
  warn period Logical20 : xbsReplacements_r4/Warning  SystemSampleTime=-1  period=1
  warn period not_valid0 : xbsReplacements_r4/Warning  SystemSampleTime=-1  period=1
  data_out : Outport  OutDataType=sfix(16)  OutScaling=2^0
  valid : Outport  Port=2  OutDataType=sfix(16)  OutScaling=2^0
  full : Outport  Port=3  OutDataType=sfix(16)  OutScaling=2^0
  %full : Outport  Port=4  OutDataType=sfix(16)  OutScaling=2^0
  wires:
  din/1 -> FIFO/1
  we/1 -> FIFO/2
  FIFO/2 -> not_valid/1
  ack/1 -> Convert2/1
  FIFO/1 -> data_out/1
  FIFO/4 -> full/1
  Inverter3/1 -> valid/1
  reset/1 -> FIFO/4, not_valid/2
  Logical2/1 -> FIFO/3, not_valid/3
  not_valid/1 -> Convert1/1
  Convert/1 -> Logical2/1
  FIFO/3 -> %full/1
  Convert1/1 -> Inverter3/1, Convert/1
  Convert2/1 -> Logical2/2

== system casper_library_accumulators/dram_vacc/ctrl_unit ==
  valid_data : Inport  OutDataType=sfix(16)  OutScaling=2^0
  sync : Inport  Port=2  OutDataType=sfix(16)  OutScaling=2^0
  en_RB_addr : Inport  Port=3  OutDataType=sfix(16)  OutScaling=2^0
  Concat1 : xbsIndex_r4/Concat  num_inputs=3  dbl_ovrd=off  block_type=concat
      settings: block_version=9.2.01
  Convert2 : xbsIndex_r4/Convert  arith_type=Unsigned  n_bits=30  bin_pt=0  quantization=Truncate  overflow=Wrap  latency=0  dbl_ovrd=off  pipeline=off  block_type=convert
      settings: xl_area=[0, 0, 0, 0, 0, 0, 0]  block_version=9.2.01
  Delay1 : xbsIndex_r4/Delay  en=off  latency=2  dbl_ovrd=off  reg_retiming=off  block_type=delay
      settings: xl_area=[0, 0, 0, 0, 0, 0, 0]  block_version=9.2.01
  Delay2 : xbsIndex_r4/Delay  en=off  latency=1  dbl_ovrd=off  reg_retiming=off  block_type=delay
      settings: xl_area=[0, 0, 0, 0, 0, 0, 0]  block_version=9.2.01
  Mux : xbsIndex_r4/Mux  inputs=2  en=off  latency=0  precision=Full  arith_type="Signed  (2's comp)"  n_bits=8  bin_pt=2  quantization=Truncate  overflow=Wrap  dbl_ovrd=off  block_type=mux
      settings: xl_area=[0, 0, 0, 0, 0, 0, 0]  block_version=9.2.01
  Mux2 : xbsIndex_r4/Mux  inputs=2  en=off  latency=0  precision=Full  arith_type="Signed  (2's comp)"  n_bits=8  bin_pt=2  quantization=Truncate  overflow=Wrap  dbl_ovrd=off  block_type=mux
      settings: xl_area=[0, 0, 0, 0, 0, 0, 0]  block_version=9.2.01
  RB_active_or_finish : Subsystem
  address_gen_vacc_DRAM : Subsystem  mask{acc_length=acc_length, valid_length=burst_length}
      mask prompts: acc_length "Accumulation length?"; valid_length "Valid period length?"
      mask init:
      | address_gen_vacc_v2_mask;
  cmd_gen : Subsystem
  latch_rb_enable : Subsystem
  negedge : Subsystem
  readback_address_dram_vacc : Subsystem  mask{acc_length=acc_length, valid_length=valid_length}
      mask prompts: acc_length "Accumulation length?"; valid_length "Valid period length?"
      mask init:
      | readback_address_dram_vacc_mask;
  warn period Delay10 : xbsReplacements_r4/Warning  SystemSampleTime=-1  period=1
  warn period Delay20 : xbsReplacements_r4/Warning  SystemSampleTime=-1  period=1
  address : Outport  OutDataType=sfix(16)  OutScaling=2^0
  cmd_tag : Outport  Port=2  OutDataType=sfix(16)  OutScaling=2^0
  RB_active : Outport  Port=3  OutDataType=sfix(16)  OutScaling=2^0
  RWn : Outport  Port=4  OutDataType=sfix(16)  OutScaling=2^0
  cmd_valid : Outport  Port=5  OutDataType=sfix(16)  OutScaling=2^0
  ready : Outport  Port=6  OutDataType=sfix(16)  OutScaling=2^0
  wires:
  latch_rb_enable/2(cmd_tag) -> Concat1/3
  Delay1/1 -> latch_rb_enable/1(sync), readback_address_dram_vacc/1(sync)  "v"
  negedge/1(out) -> latch_rb_enable/3(negedge)
  latch_rb_enable/1(inc_addr_en) -> RB_active_or_finish/1(enable_rb_addr), readback_address_dram_vacc/2(en)
  readback_address_dram_vacc/1(readback_addr) -> Mux2/3
  valid_data/1 -> cmd_gen/1(valid_data)
  cmd_gen/6(rb_addr_en) -> negedge/1(in), Concat1/1, Mux2/1
  cmd_gen/5(ready) -> ready/1
  cmd_gen/4(cmd_valid) -> cmd_valid/1
  cmd_gen/3(RWn) -> Mux/1, RWn/1
  RB_active_or_finish/1(rb_active) -> RB_active/1
  Mux2/1 -> address/1, Convert2/1
  en_RB_addr/1 -> latch_rb_enable/2(rb_addr_enable)
  Delay2/1 -> address_gen_vacc_DRAM/1(sync)
  Concat1/1 -> cmd_tag/1
  Convert2/1 -> Concat1/2
  cmd_gen/2(wr_addr_en) -> address_gen_vacc_DRAM/3(write_en)
  cmd_gen/1(re_addr_en) -> address_gen_vacc_DRAM/2(read_en)
  Mux/1 -> Mux2/2
  address_gen_vacc_DRAM/2(read_addr) -> Mux/3
  address_gen_vacc_DRAM/1(write_addr) -> Mux/2
  sync/1 -> Delay2/1, RB_active_or_finish/2(sync), Delay1/1, cmd_gen/2(sync)
